simulink model "Lettuce_System_Simulation"  (R2019a)
settings: Solver=VariableStepAuto  StartTime=0.0  StopTime=60  RelTol=1e-3
libraries: sh_lib x6, nesl_utility x6, fl_lib x4
settings Model: Creator=erwin  LastModifiedBy=erwin

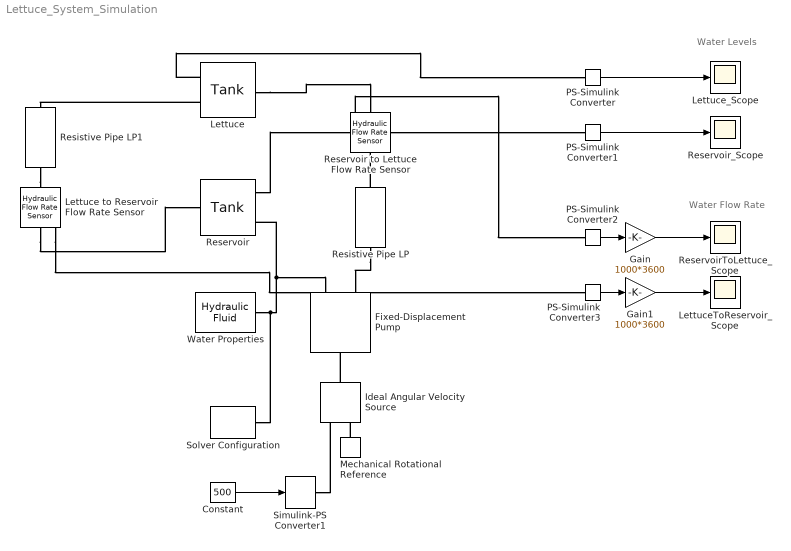
== system Lettuce_System_Simulation ==
  note: Water Flow Rate
  note: Water Levels
  " Water Properties" : sh_lib/Hydraulic Utilities/Hydraulic Fluid  DataSource=1  SelFluid=24  SysTemp=60  TrapAir=0.005  ViscDerFactor=1  range_error=2
      settings: SourceProductName=Simscape Fluids
  Constant : Constant  Value=500
  Fixed-Displacement Pump : sh_lib/Pumps and Motors/Fixed-Displacement Pump  D=30 cm^3/rev  loss_spec=1  w_nominal=188 rad/s  pr_nominal=100e5 Pa  visc_nominal=18 cSt  dens_nominal=900 kg/m^3  efficiency_vol=0.92  no_load_torque=0.05 N*m  torque_pressure_coeff=0.6e-6 N*m/Pa  p_diff_eff_TLU=[100000, 1000000, 2000000] Pa  omega_eff_TLU=[25, 50, 100, 200, 300, 400] rad/s  vol_eff_TLU=[.816, .908, .954, .977, .981, .984; .325, .663, .831, .916, .925, .946; .137, .568, .78, .892, .893, .91]  mech_eff_TLU=[.996, .996, .996, .996, .996, .996; .988, .989, .989, .989, .989, .99; .981, .981, .982, .982, .983, .984]  p_diff_loss_TLU=[100000, 1000000, 2000000] Pa  omega_loss_TLU=[25, 50, 100, 200, 300, 400] rad/s  vol_loss_TLU=[.023, .023, .023, .023, .0285, .032; .0844, .0842, .0845, .084, .1125, .108; .1079, .108, .11, .108, .1605, .18] * 1e-3 m^3/s  mech_loss_TLU=[.002, .002, .002, .002, .002, .002; .0607, .0556, .0556, .0556, .0556, .0505; .1937, .1937, .1833, .1833, .1729, .1626] N*m  pressure_threshold=1e5 Pa  omega_threshold=10 rad/s  quadrant_check=0  pressure_check=0  min_valid_pressure=0 Pa  vol_eff_min=1e-3  vol_eff_max=1  mech_eff_min=1e-3  mech_eff_max=1
      settings: SourceProductName=Simscape Fluids  SourceProductBaseCode=SH
  Gain : Gain  Gain=1000*3600
  Gain1 : Gain  Gain=1000*3600
  Ideal Angular Velocity Source : fl_lib/Mechanical/Mechanical Sources/Ideal Angular Velocity Source
  Lettuce : sh_lib/Low-Pressure Blocks/Tank  press=0 Pa  level_spec=1  tank_area=0.8 m^2  fluid_volume_tab=[0, .0028, .0065, .0114, .0176, .0252, .0344, .0436, .0512, .0574, .0623, .066, .0688, .0707, .072, .0727] m^3  fluid_level_tab=[0, .02, .04, .06, .08, .1, .12, .14, .16, .18, .2, .22, .24, .26, .28, .3] m  interp_method=1  extrap_method=1  pipe_diam=0.02 m  loss_coeff=1.2  g=9.80665 m/s^2  min_level=1e-3 m  fluid_level_check=1  volume_specify=on  volume_priority=High  volume=2 l  volume_nominal_specify=off  volume_nominal_unit=l  volume_nominal_value=1  level_specify=off  level_priority=None  level=0.025 m  level_nominal_specify=off  level_nominal_unit=m  level_nominal_value=1  pipe_diam_A=1 in  loss_coeff_A=1.2  height_B=0.8 m  pipe_diam_B=1 in  loss_coeff_B=1.2  height_C=0.8 m  pipe_diam_C=0.02 m  loss_coeff_C=1.2
      settings: SourceProductName=Simscape Fluids  SourceProductBaseCode=SH
  Lettuce to Reservoir Flow Rate Sensor : fl_lib/Hydraulic/Hydraulic Sensors/Hydraulic Flow Rate Sensor
      settings: SourceProductName=Simscape
  LettuceToReservoir_Scope : Scope
  Lettuce_Scope : Scope
  Mechanical Rotational Reference : fl_lib/Mechanical/Rotational Elements/Mechanical Rotational Reference
  PS-Simulink Converter : nesl_utility/PS-Simulink Converter  PhysicalDomain=network_engine_domain  SubClassName=ps_output  LeftPortType=input  RightPortType=output  PseudoPeriodic=off  Frequencies=[]  Unit=l  AffineConversion=off
  PS-Simulink Converter1 : nesl_utility/PS-Simulink Converter  PhysicalDomain=network_engine_domain  SubClassName=ps_output  LeftPortType=input  RightPortType=output  PseudoPeriodic=off  Frequencies=[]  Unit=l  AffineConversion=off
  PS-Simulink Converter2 : nesl_utility/PS-Simulink Converter  PhysicalDomain=network_engine_domain  SubClassName=ps_output  LeftPortType=input  RightPortType=output  PseudoPeriodic=off  Frequencies=[]  Unit=m^3/s  AffineConversion=on
  PS-Simulink Converter3 : nesl_utility/PS-Simulink Converter  PhysicalDomain=network_engine_domain  SubClassName=ps_output  LeftPortType=input  RightPortType=output  PseudoPeriodic=off  Frequencies=[]  Unit=m^3/s  AffineConversion=on
  Reservoir : sh_lib/Low-Pressure Blocks/Tank  press=0 Pa  level_spec=1  tank_area=0.8 m^2  fluid_volume_tab=[0, .0028, .0065, .0114, .0176, .0252, .0344, .0436, .0512, .0574, .0623, .066, .0688, .0707, .072, .0727] m^3  fluid_level_tab=[0, .02, .04, .06, .08, .1, .12, .14, .16, .18, .2, .22, .24, .26, .28, .3] m  interp_method=1  extrap_method=1  pipe_diam=0.02 m  loss_coeff=1.2  g=9.80665 m/s^2  min_level=1e-3 m  fluid_level_check=1  volume_specify=on  volume_priority=High  volume=10 l  volume_nominal_specify=off  volume_nominal_unit=l  volume_nominal_value=1  level_specify=off  level_priority=None  level=0.025 m  level_nominal_specify=off  level_nominal_unit=m  level_nominal_value=1  pipe_diam_A=1 in  loss_coeff_A=1.2  height_B=0.8 m  pipe_diam_B=1 in  loss_coeff_B=1.2  height_C=0.8 m  pipe_diam_C=0.02 m  loss_coeff_C=1.2
      settings: SourceProductName=Simscape Fluids  SourceProductBaseCode=SH
  Reservoir to Lettuce Flow Rate Sensor : fl_lib/Hydraulic/Hydraulic Sensors/Hydraulic Flow Rate Sensor
      settings: SourceProductName=Simscape
  ReservoirToLettuce_Scope : Scope
  Reservoir_Scope : Scope
  Resistive Pipe LP : sh_lib/Low-Pressure Blocks/Resistive Pipe LP  cs_type=1  d_in=0.01 m  area=1e-4 m^2  D_h=1.12e-2 m  s_factor=64  length=5 m  length_ad=1 m  roughness=15e-6 m  Re_lam=2000  Re_turb=4000  elevation_A=0 m  elevation_B=0.3 m  g=9.80665 m/s^2  pressure_drop_specify=off  pressure_drop_priority=None  pressure_drop=0 Pa  pressure_drop_nominal_specify=off  pressure_drop_nominal_unit=Pa  pressure_drop_nominal_value=1  flow_rate_specify=off  flow_rate_priority=None  flow_rate=10 lpm  flow_rate_nominal_specify=off  flow_rate_nominal_unit=m^3/s  flow_rate_nominal_value=1
      settings: SourceProductName=Simscape Fluids  SourceProductBaseCode=SH
  Resistive Pipe LP1 : sh_lib/Low-Pressure Blocks/Resistive Pipe LP  cs_type=1  d_in=0.01 m  area=1e-4 m^2  D_h=1.12e-2 m  s_factor=64  length=5 m  length_ad=1 m  roughness=15e-6 m  Re_lam=2000  Re_turb=4000  elevation_A=300 cm  elevation_B=0 m  g=9.80665 m/s^2  pressure_drop_specify=off  pressure_drop_priority=None  pressure_drop=0 Pa  pressure_drop_nominal_specify=off  pressure_drop_nominal_unit=Pa  pressure_drop_nominal_value=1  flow_rate_specify=off  flow_rate_priority=None  flow_rate=10 lpm  flow_rate_nominal_specify=off  flow_rate_nominal_unit=m^3/s  flow_rate_nominal_value=1
      settings: SourceProductName=Simscape Fluids  SourceProductBaseCode=SH
  Simulink-PS Converter1 : nesl_utility/Simulink-PS Converter  PhysicalDomain=network_engine_domain  SubClassName=ps_input  LeftPortType=input  RightPortType=output  PseudoPeriodic=off  Frequencies=[]  NoiseDistribution=none  NoiseParameters=[]  Unit=rpm  AffineConversion=off  FilteringAndDerivatives=zero  SimscapeFilterOrder=1  InputFilterTimeConstant=.001  UdotUserProvided=0
  Solver Configuration : nesl_utility/Solver Configuration  PhysicalDomain=network_engine_domain  SubClassName=solver  LeftPortType=input  RightPortType=generic  Tones=[]  Harmonics=[]  SimulateNoise=off  Profile=off  UseLocalSampling=off  EnableSwitchedLinearOptims=on  FrequencyDomain=off  UseCCode=off  RelTol=0.001  AbsTol=1e-06  MinStep=1e-09  ToWorkspace=off  RevertToSquareIcSolve=off  NumHomotopyIterations=100  PhasorMode=off  PhasorModeNumHarmonics=1  DoDC=off  ResidualTolerance=1e-9  UseLocalSolver=off  LocalSolverChoice=NE_BACKWARD_EULER_ADVANCER  LocalSolverSampleTime=.001  DoFixedCost=off  MaxNonlinIter=3  MaxModeIter=2  LinearAlgebra=auto  EquationFormulation=NE_TIME_EF  DelaysMemoryBudget=1024  AutomaticFiltering=on  FilteringTimeConstant=0.001  PartitionStorageMethod=AS_NEEDED  PartitionMemoryBudget=1024  PartitionMethod=FAST
  wires:
  PS-Simulink Converter/1 -> Lettuce_Scope/1
  PS-Simulink Converter1/1 -> Reservoir_Scope/1
  PS-Simulink Converter2/1 -> Gain/1
  Constant/1 -> Simulink-PS Converter1/1
  Gain/1 -> ReservoirToLettuce_Scope/1
  PS-Simulink Converter3/1 -> Gain1/1
  Gain1/1 -> LettuceToReservoir_Scope/1
  connections:
  " Water Properties"/RConn1 -- Fixed-Displacement Pump/RConn2 -- Reservoir/RConn2 -- Solver Configuration/RConn1
  Lettuce/RConn1 -- PS-Simulink Converter/LConn1
  Reservoir/RConn1 -- PS-Simulink Converter1/LConn1
  Reservoir to Lettuce Flow Rate Sensor/RConn1 -- PS-Simulink Converter2/LConn1
  Lettuce to Reservoir Flow Rate Sensor/RConn2 -- Reservoir/LConn1
  Lettuce to Reservoir Flow Rate Sensor/RConn1 -- PS-Simulink Converter3/LConn1
  Resistive Pipe LP1/RConn1 -- Lettuce to Reservoir Flow Rate Sensor/LConn1
  Resistive Pipe LP/RConn1 -- Reservoir to Lettuce Flow Rate Sensor/LConn1
  Mechanical Rotational Reference/LConn1 -- Ideal Angular Velocity Source/RConn2
  Simulink-PS Converter1/RConn1 -- Ideal Angular Velocity Source/RConn1
  Ideal Angular Velocity Source/LConn1 -- Fixed-Displacement Pump/LConn1
  Resistive Pipe LP/LConn1 -- Fixed-Displacement Pump/RConn1
  Lettuce/LConn1 -- Reservoir to Lettuce Flow Rate Sensor/RConn2
  Lettuce/RConn2 -- Resistive Pipe LP1/LConn1
